simulink model "i_node2"  (R2012b)
settings: Solver=FixedStepDiscrete  SolverMode=SingleTasking  StartTime=0.0  StopTime=inf  RelTol=1e-3
model workspace (MAT data in the model file):
  Param = Simulink.Parameter
  Param.DataType = 'auto'
libraries: dspsigops x4, simulink x1
settings Model: Creator=andreas  LastModifiedBy=andreas
settings DataIOCC: SaveOutput=off  SignalLogging=off  SaveTime=off
settings OptimizationCC: InlineParams=on
settings DebuggingCC: AlgebraicLoopMsg=error  SingleTaskRateTransMsg=error

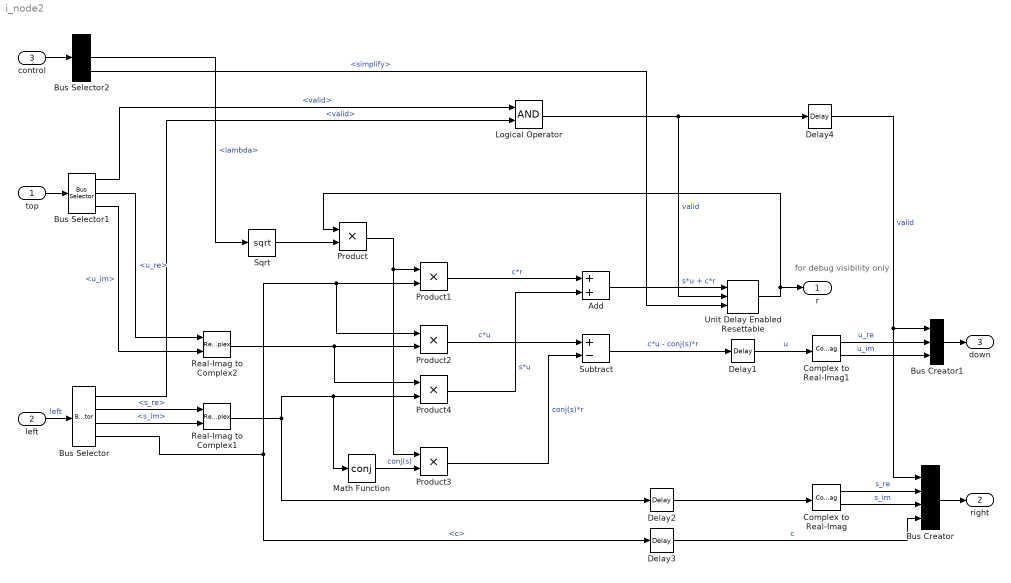
== system i_node2 ==
  note: for debug visibility only
  top : Inport  OutDataTypeStr=Bus: vbus
      settings: SignalType=complex
  left : Inport  Port=2  OutDataTypeStr=Bus: hbus
      settings: SignalType=complex
  control : Inport  Port=3  OutDataTypeStr=Bus: cbus
  Add : Sum
  Bus Creator : BusCreator
  Bus Creator1 : BusCreator  Inputs=3
  Bus Selector : BusSelector  OutputSignals=valid,s_re,s_im,c
  Bus Selector1 : BusSelector  OutputSignals=valid,u_re,u_im
  Bus Selector2 : BusSelector  OutputSignals=boundary_ic,lambda,simplify
  Complex to Real-Imag : ComplexToRealImag
  Complex to Real-Imag1 : ComplexToRealImag
  Delay{1..4} (4 alike) : dspsigops/Delay  InputProcessing=Columns as channels (frame based)  dly_unit=Samples  delay=1  ic_detail=off  dif_ic_for_ch=off  dif_ic_for_dly=off  ic=0  reset_popup=None
  Logical Operator : Logic  AllPortsSameDT=off  OutDataTypeStr=boolean
  Math Function : Math  Operator=conj  SaturateOnIntegerOverflow=on
  Product{,1..4} (5 alike) : Product  RndMeth=Zero
  Real-Imag to Complex1 : RealImagToComplex
  Real-Imag to Complex2 : RealImagToComplex
  Sqrt : Sqrt  SaturateOnIntegerOverflow=on
  Subtract : Sum  Inputs=+-
  Unit Delay Enabled Resettable : simulink/Additional Math & Discrete/Additional Discrete/Unit Delay Enabled Resettable  vinit=complex(0,0)  tsamp=-1
  r : Outport
  right : Outport  Port=2  OutDataTypeStr=Bus: hbus
  down : Outport  Port=3  OutDataTypeStr=Bus: vbus
  wires:
  Real-Imag to Complex1/1 -> Math Function/1, Product4/2, Delay2/1
  Product/1 -> Product3/1, Product1/1
  Product1/1 -> Add/1  "c*r"
  Real-Imag to Complex2/1 -> Product4/1, Product2/2
  Math Function/1 -> Product3/2  "conj(s)"
  Product3/1 -> Subtract/2  "conj(s)*r"
  Product4/1 -> Add/2  "s*u"
  Product2/1 -> Subtract/1  "c*u"
  Add/1 -> Unit Delay Enabled Resettable/1  "s*u + c*r"
  Subtract/1 -> Delay1/1  "c*u - conj(s)*r"
  Complex to Real-Imag1/1 -> Bus Creator1/2  "u_re"
  Delay2/1 -> Complex to Real-Imag/1
  Sqrt/1 -> Product/2
  Logical Operator/1 -> Delay4/1, Unit Delay Enabled Resettable/2  "valid"
  Bus Selector1/3 -> Real-Imag to Complex2/2  "<u_im>"
  Complex to Real-Imag/1 -> Bus Creator/2  "s_re"
  Complex to Real-Imag/2 -> Bus Creator/3  "s_im"
  Delay3/1 -> Bus Creator/4  "c"
  Bus Selector1/1 -> Logical Operator/1  "<valid>"
  Bus Creator/1 -> right/1
  Bus Selector/1 -> Logical Operator/2  "<valid>"
  Bus Selector/2 -> Real-Imag to Complex1/1  "<s_re>"
  Bus Selector/3 -> Real-Imag to Complex1/2  "<s_im>"
  Bus Selector/4 -> Product2/1, Product1/2, Delay3/1  "<c>"
  left/1 -> Bus Selector/1  "left"
  Bus Creator1/1 -> down/1
  Complex to Real-Imag1/2 -> Bus Creator1/3  "u_im"
  Delay1/1 -> Complex to Real-Imag1/1  "u"
  Bus Selector1/2 -> Real-Imag to Complex2/1  "<u_re>"
  top/1 -> Bus Selector1/1
  Delay4/1 -> Bus Creator1/1, Bus Creator/1  "valid"
  control/1 -> Bus Selector2/1
  Bus Selector2/2 -> Sqrt/1  "<lambda>"
  Unit Delay Enabled Resettable/1 -> Product/1, r/1
  Bus Selector2/3 -> Unit Delay Enabled Resettable/3  "<simplify>"
